simulink model "adcconv_subpub"  (R2019b)
settings: Solver=FixedStepDiscrete  StartTime=0.0  StopTime=Inf  FixedStep=0.1  RelTol=1e-3  EnableMultiTasking=on
libraries: robotlib x3
settings Model: Creator=The MathWorks, Inc.  LastModifiedBy=mackst
settings DataIOCC: LimitDataPoints=on  SaveFormat=Array  ReturnWorkspaceOutputs=off
settings OptimizationCC: LifeSpan=Inf  MaxStackSize=64
settings DebuggingCC: SolverPrmCheckMsg=warning  AllowSymbolicDim=off  SFUnexpectedBacktrackingDiag=warning  SFNoUnconditionalDefaultTransitionDiag=warning  SFExecutionAtInitializationDiag=none  ArithmeticOperatorsInVariantConditions=warning
settings HardwareCC: ProdBitPerPointer=32  ProdBitPerSizeT=32  ProdBitPerPtrDiffT=32  ProdLargestAtomicFloat=None  ProdIntDivRoundTo=Undefined  ProdEndianess=Unspecified  ProdWordSize=32  ProdHWDeviceType=Generic->Unspecified (assume 32-bit Generic)  TargetHWDeviceType=Generic->Unspecified (assume 32-bit Generic)  UseEmbeddedCoderFeatures=off
settings ModelReferenceCC: PropagateSignalLabelsOutOfModel=off
settings SFSimCC: SimUseLocalCustomCode=off  CustomCodeUndefinedFunction=UseInterfaceOnly
settings RTWCC: SystemTargetFile=ert.tlc  HardwareBoard=Robot Operating System (ROS)  TemplateMakefile=ert_default_tmf  RTWUseLocalCustomCode=off  Toolchain=Catkin  TargetLang=C++
settings CodeAppCC: StateflowObjectComments=on
settings ERTTargetCC: MultiwordLength=2048  ERTCustomFileBanners=off  MultiInstanceERTCode=on  CodeInterfacePackaging=C++ class  SupportContinuousTime=on  SupportNonInlinedSFcns=on  RemoveResetFunc=off  SupportVariableSizeSignals=on  ModelStepFunctionPrototypeControlCompliant=off  RootIOFormat=Structure reference  ConvertIfToSwitch=off  SuppressUnreachableDefaultCases=off
settings ConfigComp: CovMetricSettings=dw  CovHtmlReporting=on  CovSaveCumulativeToWorkspaceVar=on  CovSaveSingleToWorkspaceVar=on  CovExternalEMLEnable=off  CovSFcnEnable=off

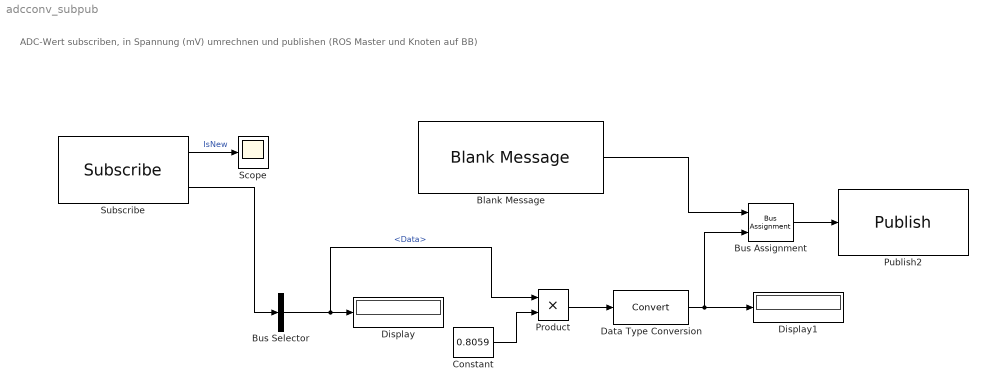
== system adcconv_subpub ==
  note: ADC-Wert subscriben, in Spannung (mV) umrechnen und publishen (ROS Master und Knoten auf BB)
  Blank Message : robotlib/Blank Message  messageClass=Message  entityType=std_msgs/Int16  messageType=std_msgs/Int16  SampleTime=-1
      settings: SourceProductName=ROS Toolbox
  Bus Assignment : BusAssignment  AssignedSignals=Data
  Bus Selector : BusSelector  OutputSignals=Data
  Constant : Constant  Value=0.8059
  Data Type Conversion : DataTypeConversion
  Display : Display
  Display1 : Display
  Product : Product
  Publish2 : robotlib/Publish  topicSource=Specify your own  topic=/adc_val_mv  messageType=std_msgs/Int16  messageQueueLength=105
      settings: SourceProductName=ROS Toolbox
  Scope : Scope
  Subscribe : robotlib/Subscribe  topicSource=Select from ROS network  topic=/adc_val  messageType=std_msgs/UInt16  sampleTime=-1  messageQueueLength=51
      settings: SourceProductName=ROS Toolbox
  wires:
  Subscribe/1 -> Scope/1  "IsNew"
  Subscribe/2 -> Bus Selector/1
  Bus Selector/1 -> Product/1, Display/1  "<Data>"
  Product/1 -> Data Type Conversion/1
  Bus Assignment/1 -> Publish2/1
  Blank Message/1 -> Bus Assignment/1
  Data Type Conversion/1 -> Bus Assignment/2, Display1/1
  Constant/1 -> Product/2
